simulink model "db4_5"  (R2018a)
settings: Solver=ode23t  StartTime=0.0  StopTime=10  RelTol=1e-7  AbsTol=1e-9
values from neighbouring files (symbols this model uses):
  Iaref = str2num(get(findobj('Tag','variable1'),'String'))    [simulaciones.m]
  Tc = str2num(get(findobj('Tag','variable6'),'String'))    [graficas_a.m]    (also in simulaciones.m = str2num(get(findobj('Tag','variable5'),'String')))
  tTc = str2num(get(findobj('Tag','variable6'),'String'))    [graficas_a.m]    (also in simulaciones.m)
settings Model: ExtModeTrigMode=oneshot  ExtModeArmWhenConnect=off  Creator=Administrador  LastModifiedBy=LAC-TELECOM-OLI-02
settings SolverCC: AutoScaleAbsTol=off
settings DataIOCC: SaveFormat=Array  SignalLoggingSaveFormat=ModelDataLogs
settings OptimizationCC: BlockReduction=off  BooleanDataType=off  ExpressionDepthLimit=2147483647  InitFltsAndDblsToZero=on  LifeSpan=inf
settings DebuggingCC: SaveWithParameterizedLinksMsg=none  UnderspecifiedInitializationDetection=Classic  MergeDetectMultiDrivingBlocksExec=none  SignalResolutionControl=TryResolveAllWithWarning  MultiTaskDSMMsg=warning  MultiTaskCondExecSysMsg=none  FcnCallInpInsideContextMsg=warning  StateNameClashWarn=warning  SFUnexpectedBacktrackingDiag=warning  SFNoUnconditionalDefaultTransitionDiag=warning  SFExecutionAtInitializationDiag=none
settings HardwareCC: ProdBitPerPointer=32  ProdBitPerSizeT=32  ProdBitPerPtrDiffT=32  ProdLargestAtomicFloat=None  ProdIntDivRoundTo=Undefined  ProdEndianess=Unspecified  ProdWordSize=32  ProdHWDeviceType=32-bit Generic  TargetUnknown=on
settings ModelReferenceCC: PropagateSignalLabelsOutOfModel=off
settings RTWCC: TemplateMakefile=grt_vc.tmf
settings CodeAppCC: StateflowObjectComments=on
settings GRTTargetCC: TargetLangStandard=C89/C90 (ANSI)  GeneratePreprocessorConditionals=Disable all  CombineOutputUpdateFcns=off  GRTInterface=on
settings ConfigComp: CovMetricSettings=dw  CovHtmlReporting=on  CovSaveCumulativeToWorkspaceVar=on  CovSaveSingleToWorkspaceVar=on  CovExternalEMLEnable=off

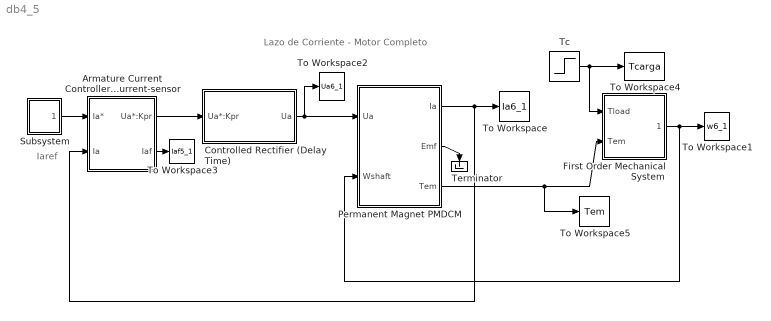
== system db4_5 ==
  note: Lazo de Corriente - Motor Completo
  note: Iaref
  Armature Current Controller (PI) with Current-sensor : Subsystem  mask(Armature Current Controller with Current-sensor){d=on, Kpi=0.008, TIi=0.027, Kti=1, Tfi=0.008}
      mask prompts: d "Zero pre-compensation"; Kpi "Current Proportional Gain:"; TIi "Current Integral Gain:"; Kti "Current-sensor Proportional Gain:"; Tfi "Current-sensor Integral Gain:"
      mask init:
      | if d==1
      | TIi_c=TIi;
      | else
      | TIi_c=0;
      | end
  Controlled Rectifier (Delay Time) : Subsystem  mask(Controlled Rectifier (Delay Time)){Tpr=0.00167, Kpr=20}
      mask prompts: Tpr "Delay Time:"; Kpr "Controlled Rectifier Proportional Gain:"
      mask help: Kpr.e(-Tpr.s)
      mask Display:
      | plot([0.5 0.6 0.6 0.75],[0.2 0.2 .8 .8 ])
      | plot([0.45 0.8 0.8 0.45 0.45],[0.15 0.15 .85 .85 0.15])
  First Order Mechanical System : Subsystem  mask(First Order Mechanical System){J=15, b=33.147, wor=0}
      mask prompts: J "Inertia [Kgm]:"; b "Friction Coeficient [Nm seg/rad]:"; wor "Speed Initial Condition [rad/sec]:"
      mask help:
      | This block solves the following differential equation:
      |
      | dW(t)/dt = - W(t)/J + (Tm -- bW(t) -- Load )/J
      | W(0)=W0
  Permanent Magnet PMDCM : Subsystem  mask(Permanent Magnet PMDCM){La=0.003, Ra=0.05, k=6.7851, ic=0}
      mask prompts: La "Armature Inductance  [Hy]:"; Ra "Armature Resistance [Ohms]:"; k "Motor Constant:"; ic "Armature Current Initial Condition [Amp]:"
  Subsystem : Subsystem
      mask Display: plot([10 20 20 40 40 60 60  80] ,[10 10 50 50 30 30 40 40 ])
  Tc : Step  Time=tTc  After=Tc  SampleTime=0
  Terminator : Terminator
  To Workspace : ToWorkspace  VariableName=Ia6_1  SampleTime=-1
  To Workspace1 : ToWorkspace  VariableName=w6_1  SampleTime=-1
  To Workspace2 : ToWorkspace  VariableName=Ua6_1  SampleTime=-1
  To Workspace3 : ToWorkspace  VariableName=Iaf5_1  SampleTime=-1
  To Workspace4 : ToWorkspace  VariableName=Tcarga  SampleTime=-1
  To Workspace5 : ToWorkspace  VariableName=Tem  SampleTime=-1
  wires:
  Subsystem/1(Out1) -> Armature Current Controller (PI) with Current-sensor/1(Ia*)
  First Order Mechanical System/1(Wshaft) -> To Workspace1/1, Permanent Magnet PMDCM/2(Wshaft)
  Permanent Magnet PMDCM/2(Emf) -> Terminator/1
  Controlled Rectifier (Delay Time)/1(Ua) -> Permanent Magnet PMDCM/1(Ua), To Workspace2/1
  Armature Current Controller (PI) with Current-sensor/1(Ua*:Kpr) -> Controlled Rectifier (Delay Time)/1(Ua*:Kpr)
  Permanent Magnet PMDCM/1(Ia) -> To Workspace/1, Armature Current Controller (PI) with Current-sensor/2(Ia)
  Armature Current Controller (PI) with Current-sensor/2(Iaf) -> To Workspace3/1
  Tc/1 -> First Order Mechanical System/1(Tload), To Workspace4/1
  Permanent Magnet PMDCM/3(Tem) -> First Order Mechanical System/2(Tem), To Workspace5/1

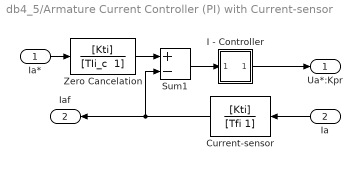
== system db4_5/Armature Current Controller (PI) with Current-sensor ==
  Ia* : Inport
  Ia : Inport  Port=2
  Current-sensor : TransferFcn  Numerator=[Kti]  Denominator=[Tfi 1]
  I - Controller : Subsystem  mask(PI Controller){P=Kpi, I=Kpi/TIi}
      mask prompts: P "Proportional:"; I "Integral:"
      mask help:
      | Enter expressions for proportional and  integral terms.
      | P+I/s
      mask Display: plot([0 0.001 5], [0 3 5])
  Sum1 : Sum  Inputs=+-  SaturateOnIntegerOverflow=on  InputSameDT=on  OutDataTypeStr=Inherit: Same as first input
  Zero Cancelation : TransferFcn  Numerator=[Kti]  Denominator="[TIi_c  1]"
  Ua*:Kpr : Outport
  Iaf : Outport  Port=2
  wires:
  Sum1/1 -> I - Controller/1(In_1)
  I - Controller/1(Out_1) -> Ua*:Kpr/1
  Ia/1 -> Current-sensor/1
  Current-sensor/1 -> Iaf/1, Sum1/2
  Zero Cancelation/1 -> Sum1/1
  Ia*/1 -> Zero Cancelation/1

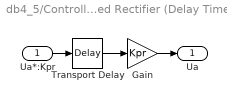
== system db4_5/Controlled Rectifier (Delay Time) ==
  Ua*:Kpr : Inport
  Gain : Gain  Gain=Kpr  SaturateOnIntegerOverflow=on  OutDataTypeStr=Inherit: Same as input  ParamDataTypeStr=Inherit: Same as input
  Transport Delay : TransportDelay  DelayTime=Tpr
  Ua : Outport
  wires:
  Ua*:Kpr/1 -> Transport Delay/1
  Transport Delay/1 -> Gain/1
  Gain/1 -> Ua/1

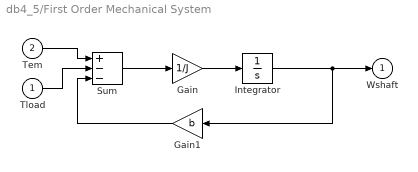
== system db4_5/First Order Mechanical System ==
  Tload : Inport
  Tem : Inport  Port=2
  Gain : Gain  Gain=1/J  SaturateOnIntegerOverflow=on  OutDataTypeStr=Inherit: Same as input  ParamDataTypeStr=Inherit: Same as input
  Gain1 : Gain  Gain=b  SaturateOnIntegerOverflow=on  OutDataTypeStr=Inherit: Same as input  ParamDataTypeStr=Inherit: Same as input
  Integrator : Integrator  InitialCondition=wor
  Sum : Sum  Inputs=+--  SaturateOnIntegerOverflow=on  InputSameDT=on  OutDataTypeStr=Inherit: Same as first input
  Wshaft : Outport
  wires:
  Integrator/1 -> Wshaft/1, Gain1/1
  Gain1/1 -> Sum/3
  Gain/1 -> Integrator/1
  Sum/1 -> Gain/1
  Tem/1 -> Sum/1
  Tload/1 -> Sum/2

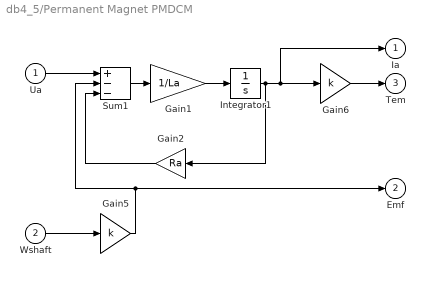
== system db4_5/Permanent Magnet PMDCM ==
  Ua : Inport
  Wshaft : Inport  Port=2
  Gain1 : Gain  Gain=1/La  SaturateOnIntegerOverflow=on  OutDataTypeStr=Inherit: Same as input  ParamDataTypeStr=Inherit: Same as input
  Gain2 : Gain  Gain=Ra  SaturateOnIntegerOverflow=on  OutDataTypeStr=Inherit: Same as input  ParamDataTypeStr=Inherit: Same as input
  Gain5 : Gain  Gain=k  SaturateOnIntegerOverflow=on  OutDataTypeStr=Inherit: Same as input  ParamDataTypeStr=Inherit: Same as input
  Gain6 : Gain  Gain=k  SaturateOnIntegerOverflow=on  OutDataTypeStr=Inherit: Same as input  ParamDataTypeStr=Inherit: Same as input
  Integrator1 : Integrator  InitialCondition=ic
  Sum1 : Sum  Inputs=+--  SaturateOnIntegerOverflow=on  InputSameDT=on  OutDataTypeStr=Inherit: Same as first input
  Ia : Outport
  Emf : Outport  Port=2
  Tem : Outport  Port=3
  wires:
  Wshaft/1 -> Gain5/1
  Gain5/1 -> Emf/1, Sum1/2
  Gain6/1 -> Tem/1
  Ua/1 -> Sum1/1
  Sum1/1 -> Gain1/1
  Gain1/1 -> Integrator1/1
  Gain2/1 -> Sum1/3
  Integrator1/1 -> Gain2/1, Ia/1, Gain6/1

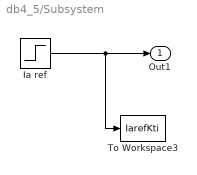
== system db4_5/Subsystem ==
  "Ia ref " : Step  Time=0  After=Iaref  SampleTime=0
  To Workspace3 : ToWorkspace  VariableName=IarefKti  SampleTime=-1
  Out1 : Outport
  wires:
  "Ia ref "/1 -> To Workspace3/1, Out1/1

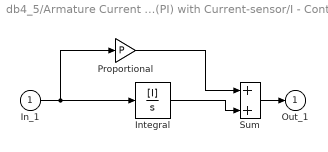
== system db4_5/Armature Current Controller (PI) with Current-sensor/I - Controller ==
  In_1 : Inport
  Integral : TransferFcn  Numerator=[I]  Denominator=[1 0]
  Proportional : Gain  Gain=P  SaturateOnIntegerOverflow=on  OutDataTypeStr=Inherit: Same as input  ParamDataTypeStr=Inherit: Same as input
  Sum : Sum  SaturateOnIntegerOverflow=on  InputSameDT=on  OutDataTypeStr=Inherit: Same as first input
  Out_1 : Outport
  wires:
  In_1/1 -> Proportional/1, Integral/1
  Sum/1 -> Out_1/1
  Integral/1 -> Sum/2
  Proportional/1 -> Sum/1
